simulink model "progetto"  (R2022b)
settings: Solver=VariableStepAuto  StartTime=0.0  StopTime=10  RelTol=1e-3
undefined symbols (not defined in the file): c, J, k_amp, k_ff, kdt, kt, kv, La, Ra
settings Model: Creator=tedoa  LastModifiedBy=tedoa

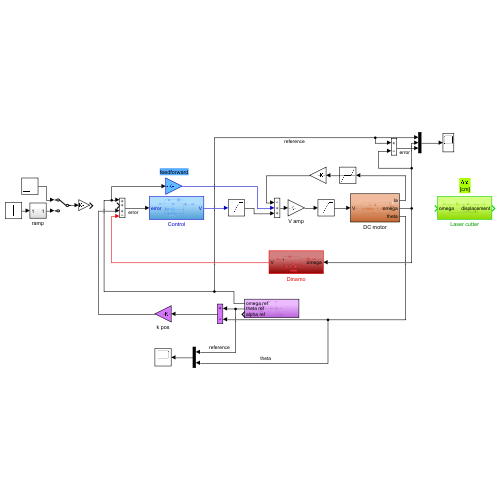
[thumbnail: Simulink's stored preview of the top-level diagram]
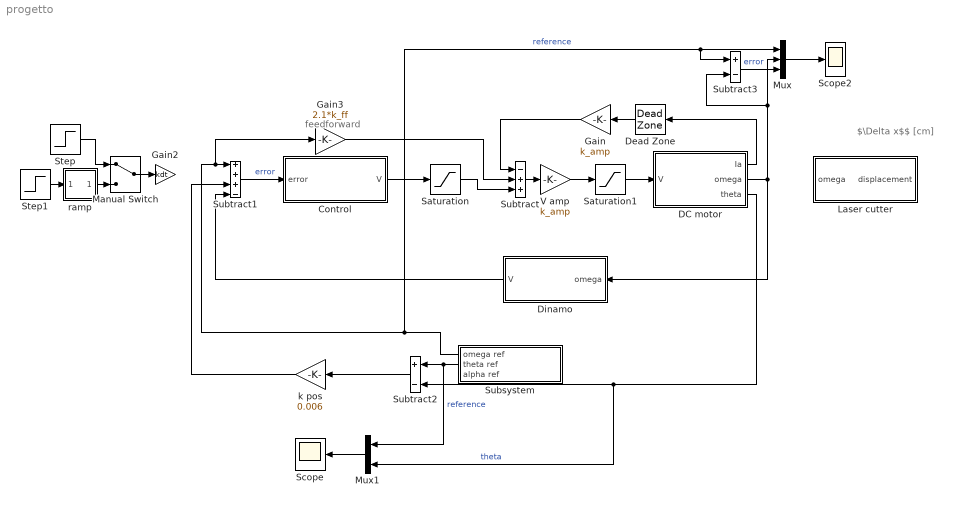
== system progetto ==
  note: $\Delta x$$
      | [cm]
  note: feedforward
  Control : Subsystem
  DC motor : Subsystem
  Dead Zone : DeadZone  LowerValue=-2.273  UpperValue=2.273
  Dinamo : Subsystem
  Gain : Gain  Gain=k_amp
  Gain2 : Gain  Gain=kdt
  Gain3 : Gain  Gain=2.1*k_ff
  Laser cutter : Subsystem
  Manual Switch : ManualSwitch
  Mux : Mux  Inputs=3
  Mux1 : Mux  Inputs=2
  Saturation : Saturate  UpperLimit=36*1.2  LowerLimit=-36*1.2
  Saturation1 : Saturate  UpperLimit=36*1.2  LowerLimit=-36*1.2
  Scope : Scope
  Scope2 : Scope
  Step : Step  After=3  SampleTime=0
  Step1 : Step  After=30  SampleTime=0
  Subsystem : Subsystem
  Subtract : Sum  Inputs=-++
  Subtract1 : Sum  Inputs=+++-
  Subtract2 : Sum  Inputs=+-
  Subtract3 : Sum  Inputs=+-
  V amp : Gain  Gain=k_amp
  k pos : Gain  Gain=0.006
  ramp : Subsystem
  wires:
  Step/1 -> Manual Switch/1
  DC motor/2(omega) -> Dinamo/1(omega), Subtract3/2, Mux/2
  Saturation/1 -> Subtract/3
  Subtract/1 -> V amp/1
  DC motor/1(Ia) -> Dead Zone/1
  Dead Zone/1 -> Gain/1
  Gain/1 -> Subtract/1
  Dinamo/1(V) -> Subtract1/4
  ramp/1(Out1) -> Manual Switch/2
  Step1/1 -> ramp/1(In1)
  V amp/1 -> Saturation1/1
  Saturation1/1 -> DC motor/1(V)
  Mux/1 -> Scope2/1
  Manual Switch/1 -> Gain2/1
  Control/1(V) -> Saturation/1
  Subtract1/1 -> Control/1(error)  "error"
  Subtract2/1 -> k pos/1
  k pos/1 -> Subtract1/3
  Subsystem/2(theta ref) -> Mux1/1, Subtract2/1  "reference"
  Subsystem/1(omega ref) -> Subtract3/1, Mux/1, Gain3/1, Subtract1/1  "reference"
  Gain3/1 -> Subtract/2
  Subtract3/1 -> Mux/3  "error"
  Mux1/1 -> Scope/1
  DC motor/3(theta) -> Mux1/2, Subtract2/2  "theta"

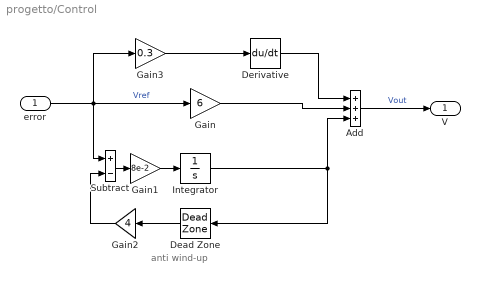
== system progetto/Control ==
  note: anti wind-up
  error : Inport
  Add : Sum  Inputs=+++
  Dead Zone : DeadZone  LowerValue=-2.32  UpperValue=2.32
  Derivative : Derivative
  Gain : Gain  Gain=6
  Gain1 : Gain  Gain=8e-2
  Gain2 : Gain  Gain=4
  Gain3 : Gain  Gain=0.3
  Integrator : Integrator  LimitOutput=on  UpperSaturationLimit=0.01  LowerSaturationLimit=-0.001
  Subtract : Sum  Inputs=+-
  V : Outport
  wires:
  Gain1/1 -> Integrator/1
  Gain/1 -> Add/2
  Integrator/1 -> Dead Zone/1, Add/3
  Subtract/1 -> Gain1/1
  error/1 -> Gain/1, Gain3/1, Subtract/1  "Vref"
  Dead Zone/1 -> Gain2/1
  Gain2/1 -> Subtract/2
  Add/1 -> V/1  "Vout"
  Gain3/1 -> Derivative/1
  Derivative/1 -> Add/1

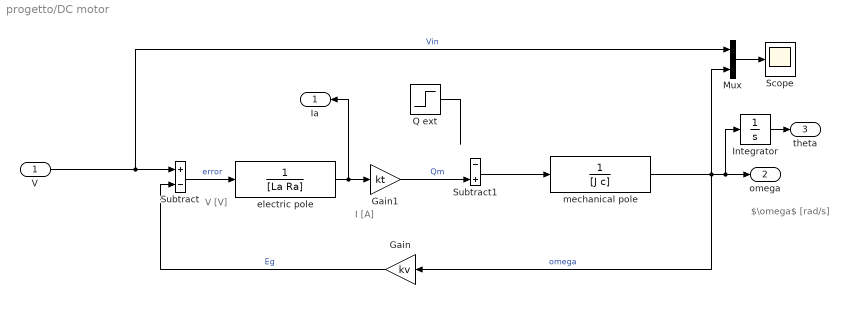
== system progetto/DC motor ==
  note: V
      | [V]
  note: I
      | [A]
  note: $\omega$
      | [rad/s]
  V : Inport
  Gain : Gain  Gain=kv
  Gain1 : Gain  Gain=kt
  Integrator : Integrator
  Mux : Mux  Inputs=2
  Q ext : Step  Time=3  After=0.03  SampleTime=0
  Scope : Scope
  Subtract : Sum  Inputs=+-
  Subtract1 : Sum  Inputs=-+
  electric pole : TransferFcn  Denominator=[La Ra]
  mechanical pole : TransferFcn  Denominator=[J c]
  Ia : Outport
  omega : Outport  Port=2
  theta : Outport  Port=3
  wires:
  electric pole/1 -> Ia/1, Gain1/1
  Gain1/1 -> Subtract1/2  "Qm"
  V/1 -> Mux/1, Subtract/1  "Vin"
  mechanical pole/1 -> Mux/2, Integrator/1, omega/1, Gain/1  "omega"
  Gain/1 -> Subtract/2  "Eg"
  Subtract/1 -> electric pole/1  "error"
  Subtract1/1 -> mechanical pole/1
  Mux/1 -> Scope/1
  Q ext/1 -> ?
  Integrator/1 -> theta/1

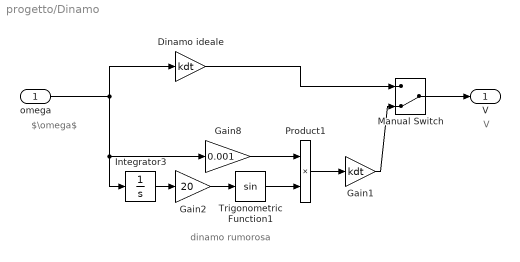
== system progetto/Dinamo ==
  note: V
  note: $\omega$
  note: dinamo rumorosa
  omega : Inport
  Dinamo ideale : Gain  Gain=kdt
  Gain1 : Gain  Gain=kdt
  Gain2 : Gain  Gain=20
  Gain8 : Gain  Gain=0.001
  Integrator3 : Integrator
  Manual Switch : ManualSwitch  CurrentSetting=0
  Product1 : Product  RndMeth=Zero
  Trigonometric Function1 : Trigonometry
  V : Outport
  wires:
  omega/1 -> Integrator3/1, Gain8/1, Dinamo ideale/1
  Dinamo ideale/1 -> Manual Switch/1
  Gain1/1 -> Manual Switch/2
  Integrator3/1 -> Gain2/1
  Gain8/1 -> Product1/1
  Gain2/1 -> Trigonometric Function1/1
  Trigonometric Function1/1 -> Product1/2
  Product1/1 -> Gain1/1
  Manual Switch/1 -> V/1

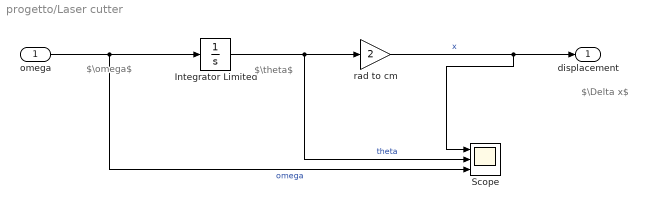
== system progetto/Laser cutter ==
  note: $\Delta x$
  note: $\theta$
  note: $\omega$
  omega : Inport
  Integrator Limited : Integrator  UpperSaturationLimit=15  LowerSaturationLimit=0
  Scope : Scope  NumInputPorts=3
  rad to cm : Gain  Gain=2
  displacement : Outport
  wires:
  omega/1 -> Integrator Limited/1, Scope/3  "omega"
  Integrator Limited/1 -> rad to cm/1, Scope/2  "theta"
  rad to cm/1 -> Scope/1, displacement/1  "x"

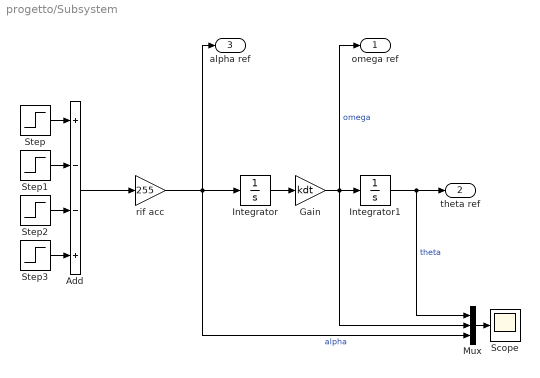
== system progetto/Subsystem ==
  Add : Sum  Inputs=+--+
  Gain : Gain  Gain=kdt
  Integrator : Integrator
  Integrator1 : Integrator
  Mux : Mux  Inputs=3
  Scope : Scope
  Step : Step  SampleTime=0
  Step1 : Step  Time=1.25  SampleTime=0
  Step2 : Step  Time=4  SampleTime=0
  Step3 : Step  Time=4.25  SampleTime=0
  rif acc : Gain  Gain=255
  omega ref : Outport
  theta ref : Outport  Port=2
  alpha ref : Outport  Port=3
  wires:
  Step/1 -> Add/1
  Step1/1 -> Add/2
  Step2/1 -> Add/3
  Step3/1 -> Add/4
  Add/1 -> rif acc/1
  rif acc/1 -> Mux/3, alpha ref/1, Integrator/1  "alpha"
  Integrator/1 -> Gain/1
  Integrator1/1 -> Mux/1, theta ref/1  "theta"
  Mux/1 -> Scope/1
  Gain/1 -> omega ref/1, Mux/2, Integrator1/1  "omega"

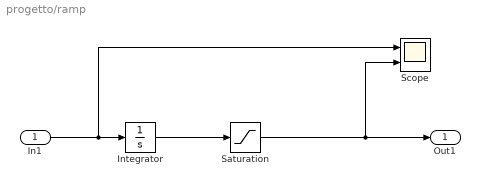
== system progetto/ramp ==
  In1 : Inport
  Integrator : Integrator
  Saturation : Saturate  UpperLimit=3  LowerLimit=0
  Scope : Scope  NumInputPorts=2
  Out1 : Outport
  wires:
  In1/1 -> Scope/1, Integrator/1
  Integrator/1 -> Saturation/1
  Saturation/1 -> Scope/2, Out1/1
